simulink model "MdInOutChk"  (R2018b)
settings: Solver=FixedStepDiscrete  StartTime=0.0  StopTime=10.0  FixedStep=0.01  RelTol=1e-3
undefined symbols (not defined in the file or in its folder): MdRspLocal2
libraries: OutRspChkLib x20
(part 1 of 2)
settings Model: Creator=sn2xws  LastModifiedBy=sn2xws
settings DataIOCC: SaveFormat=StructureWithTime
settings OptimizationCC: DefaultParameterBehavior=Inlined  EnhancedBackFolding=on  PassReuseOutputArgsAs=Individual arguments  ZeroExternalMemoryAtStartup=off  ZeroInternalMemoryAtStartup=off  OptimizeBlockOrder=speed  DifferentSizesBufferReuse=on  OptimizationCustomize=off
settings DebuggingCC: ParameterTunabilityLossMsg=error
settings ModelReferenceCC: ModelReferenceNumInstancesAllowed=Single
settings SFSimCC: MATLABDynamicMemAlloc=off
settings RTWCC: SystemTargetFile=autosar.tlc  GenCodeOnly=on  TemplateMakefile=ert_default_tmf  Description=AUTOSAR  GenerateReport=on  IncludeHyperlinkInReport=on  LaunchReport=on  GenerateTraceInfo=on  GenerateTraceReport=on  GenerateTraceReportSl=on  GenerateTraceReportSf=on  GenerateTraceReportEml=on
settings CodeAppCC: ForceParamTrailComments=on  IgnoreCustomStorageClasses=off  OperatorAnnotations=on  SimulinkDataObjDesc=on  SFDataObjDesc=on  InsertBlockDesc=on
settings STFCustomTargetCC: TargetLangStandard=C99 (ISO)  MultiwordLength=256  ParMdlRefBuildCompliant=on  CompOptLevelCompliant=on  IncludeMdlTerminateFcn=off  CombineOutputUpdateFcns=on  SuppressErrorStatus=on  ERTCustomFileBanners=on  SupportNonFinite=off  SupportComplex=off  SupportContinuousTime=off  SupportNonInlinedSFcns=off  RemoveResetFunc=on  MATLABClassNameForMDSCustomization=Simulink.SoftwareTarget.ERTCustomization  AutosarCompliant=on  UseToolchainInfoCompliant=on  LookupTableObjectStructAxisOrder=2,1,3,4,...  LUTObjectStructOrderEvenSpacing=Size,Table,Breakpoints  SystemTargetFile=autosar.tlc
settings ERTTargetCC: TargetLangStandard=C99 (ISO)  ConcurrentExecutionCompliant=off  IncludeMdlTerminateFcn=off  SuppressErrorStatus=on  SupportNonFinite=off  SupportComplex=off  ModelStepFunctionPrototypeControlCompliant=off  CPPClassGenCompliant=off  AutosarCompliant=on  LookupTableObjectStructAxisOrder=2,1,3,4,...  LUTObjectStructOrderEvenSpacing=Size,Table,Breakpoints  InlinedParameterPlacement=NonHierarchical  ERTCustomFileTemplate=example_file_process.tlc

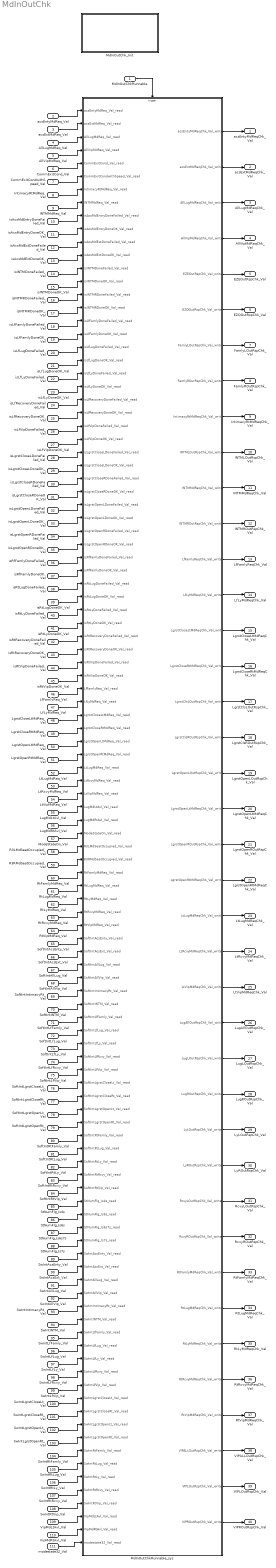
== system MdInOutChk ==
  MdInOutChkRunnable : Inport  SampleTime=0.01  OutputFunctionCall=on
  acsEntyMdReq_Val : Inport  Port=2  OutDataTypeStr=boolean  PortDimensions=1
  acsExtMdReq_Val : Inport  Port=3  OutDataTypeStr=boolean  PortDimensions=1
  AllLugMdReq_Val : Inport  Port=4  OutDataTypeStr=boolean  PortDimensions=1
  AllVipMdReq_Val : Inport  Port=5  OutDataTypeStr=boolean  PortDimensions=1
  CommExitCond_Val : Inport  Port=6  OutDataTypeStr=boolean  PortDimensions=1
  CommExitCondwithSpeed_Val : Inport  Port=7  OutDataTypeStr=boolean  PortDimensions=1
  IntimacyRtMdReq_Val : Inport  Port=8  OutDataTypeStr=boolean  PortDimensions=1
  INTMMdReq_Val : Inport  Port=9  OutDataTypeStr=boolean  PortDimensions=1
  isAcsMdEntryDoneFailed_Val : Inport  Port=10  OutDataTypeStr=boolean  PortDimensions=1
  isAcsMdEntryDoneOK_Val : Inport  Port=11  OutDataTypeStr=boolean  PortDimensions=1
  isAcsMdExtDoneFailed_Val : Inport  Port=12  OutDataTypeStr=boolean  PortDimensions=1
  isAcsMdExtDoneOK_Val : Inport  Port=13  OutDataTypeStr=boolean  PortDimensions=1
  isINTMDoneFailed_Val : Inport  Port=14  OutDataTypeStr=boolean  PortDimensions=1
  isINTMDoneOK_Val : Inport  Port=15  OutDataTypeStr=boolean  PortDimensions=1
  isINTMRDoneFailed_Val : Inport  Port=16  OutDataTypeStr=boolean  PortDimensions=1
  isINTMRDoneOK_Val : Inport  Port=17  OutDataTypeStr=boolean  PortDimensions=1
  isLfFamlyDoneFailed_Val : Inport  Port=18  OutDataTypeStr=boolean  PortDimensions=1
  isLfFamlyDoneOK_Val : Inport  Port=19  OutDataTypeStr=boolean  PortDimensions=1
  isLfLugDoneFailed_Val : Inport  Port=20  OutDataTypeStr=boolean  PortDimensions=1
  isLfLugDoneOK_Val : Inport  Port=21  OutDataTypeStr=boolean  PortDimensions=1
  isLfLyDoneFailed_Val : Inport  Port=22  OutDataTypeStr=boolean  PortDimensions=1
  isLfLyDoneOK_Val : Inport  Port=23  OutDataTypeStr=boolean  PortDimensions=1
  isLfRecoveryDoneFailed_Val : Inport  Port=24  OutDataTypeStr=boolean  PortDimensions=1
  isLfRecoveryDoneOK_Val : Inport  Port=25  OutDataTypeStr=boolean  PortDimensions=1
  isLfVipDoneFailed_Val : Inport  Port=26  OutDataTypeStr=boolean  PortDimensions=1
  isLfVipDoneOK_Val : Inport  Port=27  OutDataTypeStr=boolean  PortDimensions=1
  isLgrstCloseLDoneFailed_Val : Inport  Port=28  OutDataTypeStr=boolean  PortDimensions=1
  isLgrstCloseLDoneOK_Val : Inport  Port=29  OutDataTypeStr=boolean  PortDimensions=1
  isLgrstCloseRDoneFailed_Val : Inport  Port=30  OutDataTypeStr=boolean  PortDimensions=1
  isLgrstCloseRDoneOK_Val : Inport  Port=31  OutDataTypeStr=boolean  PortDimensions=1
  isLgrstOpenLDoneFailed_Val : Inport  Port=32  OutDataTypeStr=boolean  PortDimensions=1
  isLgrstOpenLDoneOK_Val : Inport  Port=33  OutDataTypeStr=boolean  PortDimensions=1
  isLgrstOpenRDoneFailed_Val : Inport  Port=34  OutDataTypeStr=boolean  PortDimensions=1
  isLgrstOpenRDoneOK_Val : Inport  Port=35  OutDataTypeStr=boolean  PortDimensions=1
  isRfFamlyDoneFailed_Val : Inport  Port=36  OutDataTypeStr=boolean  PortDimensions=1
  isRfFamlyDoneOK_Val : Inport  Port=37  OutDataTypeStr=boolean  PortDimensions=1
  isRtLugDoneFailed_Val : Inport  Port=38  OutDataTypeStr=boolean  PortDimensions=1
  isRtLugDoneOK_Val : Inport  Port=39  OutDataTypeStr=boolean  PortDimensions=1
  isRtLyDoneFailed_Val : Inport  Port=40  OutDataTypeStr=boolean  PortDimensions=1
  isRtLyDoneOK_Val : Inport  Port=41  OutDataTypeStr=boolean  PortDimensions=1
  isRtRecoveryDoneFailed_Val : Inport  Port=42  OutDataTypeStr=boolean  PortDimensions=1
  isRtRecoveryDoneOK_Val : Inport  Port=43  OutDataTypeStr=boolean  PortDimensions=1
  isRtVipDoneFailed_Val : Inport  Port=44  OutDataTypeStr=boolean  PortDimensions=1
  isRtVipDoneOK_Val : Inport  Port=45  OutDataTypeStr=boolean  PortDimensions=1
  LfFamlyReq_Val : Inport  Port=46  OutDataTypeStr=boolean  PortDimensions=1
  LfLyMdReq_Val : Inport  Port=47  OutDataTypeStr=boolean  PortDimensions=1
  LgrstCloseLtMdReq_Val : Inport  Port=48  OutDataTypeStr=boolean  PortDimensions=1
  LgrstCloseRtMdReq_Val : Inport  Port=49  OutDataTypeStr=boolean  PortDimensions=1
  LgrstOpenLtMdReq_Val : Inport  Port=50  OutDataTypeStr=boolean  PortDimensions=1
  LgrstOpenRtMdReq_Val : Inport  Port=51  OutDataTypeStr=boolean  PortDimensions=1
  LtLugMdReq_Val : Inport  Port=52  OutDataTypeStr=boolean  PortDimensions=1
  LtRcvyMdReq_Val : Inport  Port=53  OutDataTypeStr=boolean  PortDimensions=1
  LtVipMdReq_Val : Inport  Port=54  OutDataTypeStr=boolean  PortDimensions=1
  LugMdLtAvl_Val : Inport  Port=55  OutDataTypeStr=boolean  PortDimensions=1
  LugMdRtAvl_Val : Inport  Port=56  OutDataTypeStr=boolean  PortDimensions=1
  ModeStateOn_Val : Inport  Port=57  OutDataTypeStr=boolean  PortDimensions=1
  R3LMdSeatOccupied_Val : Inport  Port=58  OutDataTypeStr=boolean  PortDimensions=1
  R3RMdSeatOccupied_Val : Inport  Port=59  OutDataTypeStr=boolean  PortDimensions=1
  RtFamlyMdReq_Val : Inport  Port=60  OutDataTypeStr=boolean  PortDimensions=1
  RtLugMdReq_Val : Inport  Port=61  OutDataTypeStr=boolean  PortDimensions=1
  RtLyMdReq_Val : Inport  Port=62  OutDataTypeStr=boolean  PortDimensions=1
  RtRcvyMdReq_Val : Inport  Port=63  OutDataTypeStr=boolean  PortDimensions=1
  RtVipMdReq_Val : Inport  Port=64  OutDataTypeStr=boolean  PortDimensions=1
  SoftIntAcsEnty_Val : Inport  Port=65  OutDataTypeStr=IntEnable  PortDimensions=1
  SoftIntAcsExt_Val : Inport  Port=66  OutDataTypeStr=IntEnable  PortDimensions=1
  SoftIntAllLug_Val : Inport  Port=67  OutDataTypeStr=IntEnable  PortDimensions=1
  SoftIntAllVip_Val : Inport  Port=68  OutDataTypeStr=IntEnable  PortDimensions=1
  SoftIntIntimacyRt_Val : Inport  Port=69  OutDataTypeStr=IntEnable  PortDimensions=1
  SoftIntINTM_Val : Inport  Port=70  OutDataTypeStr=IntEnable  PortDimensions=1
  SoftIntLfFamly_Val : Inport  Port=71  OutDataTypeStr=IntEnable  PortDimensions=1
  SoftIntLfLug_Val : Inport  Port=72  OutDataTypeStr=IntEnable  PortDimensions=1
  SoftIntLfLy_Val : Inport  Port=73  OutDataTypeStr=IntEnable  PortDimensions=1
  SoftIntLfRcvy_Val : Inport  Port=74  OutDataTypeStr=IntEnable  PortDimensions=1
  SoftIntLfVip_Val : Inport  Port=75  OutDataTypeStr=IntEnable  PortDimensions=1
  SoftIntLgrstCloseLt_Val : Inport  Port=76  OutDataTypeStr=IntEnable  PortDimensions=1
  SoftIntLgrstCloseRt_Val : Inport  Port=77  OutDataTypeStr=IntEnable  PortDimensions=1
  SoftIntLgrstOpenLt_Val : Inport  Port=78  OutDataTypeStr=IntEnable  PortDimensions=1
  SoftIntLgrstOpenRt_Val : Inport  Port=79  OutDataTypeStr=IntEnable  PortDimensions=1
  SoftIntRtFamly_Val : Inport  Port=80  OutDataTypeStr=IntEnable  PortDimensions=1
  SoftIntRtLug_Val : Inport  Port=81  OutDataTypeStr=IntEnable  PortDimensions=1
  SoftIntRtLy_Val : Inport  Port=82  OutDataTypeStr=IntEnable  PortDimensions=1
  SoftIntRtRcvy_Val : Inport  Port=83  OutDataTypeStr=IntEnable  PortDimensions=1
  SoftIntRtVip_Val : Inport  Port=84  OutDataTypeStr=IntEnable  PortDimensions=1
  StNumFlg_Is4s : Inport  Port=85  OutDataTypeStr=boolean  PortDimensions=1
  StNumFlg_Is6s : Inport  Port=86  OutDataTypeStr=boolean  PortDimensions=1
  StNumFlg_Is6s7s : Inport  Port=87  OutDataTypeStr=boolean  PortDimensions=1
  StNumFlg_Is7s : Inport  Port=88  OutDataTypeStr=boolean  PortDimensions=1
  SwIntAcsEnty_Val : Inport  Port=89  OutDataTypeStr=IntEnable  PortDimensions=1
  SwIntAcsExt_Val : Inport  Port=90  OutDataTypeStr=IntEnable  PortDimensions=1
  SwIntAllLug_Val : Inport  Port=91  OutDataTypeStr=IntEnable  PortDimensions=1
  SwIntAllVip_Val : Inport  Port=92  OutDataTypeStr=IntEnable  PortDimensions=1
  SwIntIntimacyRt_Val : Inport  Port=93  OutDataTypeStr=IntEnable  PortDimensions=1
  SwIntINTM_Val : Inport  Port=94  OutDataTypeStr=IntEnable  PortDimensions=1
  SwIntLfFamly_Val : Inport  Port=95  OutDataTypeStr=IntEnable  PortDimensions=1
  SwIntLfLug_Val : Inport  Port=96  OutDataTypeStr=IntEnable  PortDimensions=1
  SwIntLfLy_Val : Inport  Port=97  OutDataTypeStr=IntEnable  PortDimensions=1
  SwIntLfRcvy_Val : Inport  Port=98  OutDataTypeStr=IntEnable  PortDimensions=1
  SwIntLfVip_Val : Inport  Port=99  OutDataTypeStr=IntEnable  PortDimensions=1
  SwIntLgrstCloseLt_Val : Inport  Port=100  OutDataTypeStr=IntEnable  PortDimensions=1
  SwIntLgrstCloseRt_Val : Inport  Port=101  OutDataTypeStr=IntEnable  PortDimensions=1
  SwIntLgrstOpenLt_Val : Inport  Port=102  OutDataTypeStr=IntEnable  PortDimensions=1
  SwIntLgrstOpenRt_Val : Inport  Port=103  OutDataTypeStr=IntEnable  PortDimensions=1
  SwIntRtFamly_Val : Inport  Port=104  OutDataTypeStr=IntEnable  PortDimensions=1
  SwIntRtLug_Val : Inport  Port=105  OutDataTypeStr=IntEnable  PortDimensions=1
  SwIntRtLy_Val : Inport  Port=106  OutDataTypeStr=IntEnable  PortDimensions=1
  SwIntRtRcvy_Val : Inport  Port=107  OutDataTypeStr=IntEnable  PortDimensions=1
  SwIntRtVip_Val : Inport  Port=108  OutDataTypeStr=IntEnable  PortDimensions=1
  VipMdLtAvl_Val : Inport  Port=109  OutDataTypeStr=boolean  PortDimensions=1
  VipMdRtAvl_Val : Inport  Port=110  OutDataTypeStr=boolean  PortDimensions=1
  modestate32_Val : Inport  Port=111  OutDataTypeStr=uint32  PortDimensions=1
  MdInOutChkRunnable_sys : Subsystem
  MdInOutChk_Init : Subsystem
  acsEntyMdReqChk_Val : Outport  OutDataTypeStr=boolean  PortDimensions=1
  acsExtMdReqChk_Val : Outport  Port=2  OutDataTypeStr=boolean  PortDimensions=1
  AllLugMdReqChk_Val : Outport  Port=3  OutDataTypeStr=boolean  PortDimensions=1
  AllVipMdReqChk_Val : Outport  Port=4  OutDataTypeStr=boolean  PortDimensions=1
  EZEOutRspChk_Val : Outport  Port=5  OutDataTypeStr=Enum: MdRspLocal2  PortDimensions=1
  EZQOutRspChk_Val : Outport  Port=6  OutDataTypeStr=Enum: MdRspLocal2  PortDimensions=1
  FamlyLOutRspChk_Val : Outport  Port=7  OutDataTypeStr=Enum: MdRspLocal2  PortDimensions=1
  FamlyROutRspChk_Val : Outport  Port=8  OutDataTypeStr=Enum: MdRspLocal2  PortDimensions=1
  IntimacyRtMdReqChk_Val : Outport  Port=9  OutDataTypeStr=boolean  PortDimensions=1
  INTMLOutRspChk_Val : Outport  Port=10  OutDataTypeStr=Enum: MdRspLocal2  PortDimensions=1
  INTMMdReqChk_Val : Outport  Port=11  OutDataTypeStr=boolean  PortDimensions=1
  INTMROutRspChk_Val : Outport  Port=12  OutDataTypeStr=Enum: MdRspLocal2  PortDimensions=1
  LfFamlyReqChk_Val : Outport  Port=13  OutDataTypeStr=boolean  PortDimensions=1
  LfLyMdReqChk_Val : Outport  Port=14  OutDataTypeStr=boolean  PortDimensions=1
  LgrstCloseLtMdReqChk_Val : Outport  Port=15  OutDataTypeStr=boolean  PortDimensions=1
  LgrstCloseRtMdReqChk_Val : Outport  Port=16  OutDataTypeStr=boolean  PortDimensions=1
  LgrstClsLOutRspChk_Val : Outport  Port=17  OutDataTypeStr=Enum: MdRspLocal2  PortDimensions=1
  LgrstClsROutRspChk_Val : Outport  Port=18  OutDataTypeStr=Enum: MdRspLocal2  PortDimensions=1
  LgrstOpenLOutRspChk_Val : Outport  Port=19  OutDataTypeStr=Enum: MdRspLocal2  PortDimensions=1
  LgrstOpenLtMdReqChk_Val : Outport  Port=20  OutDataTypeStr=boolean  PortDimensions=1
  LgrstOpenROutRspChk_Val : Outport  Port=21  OutDataTypeStr=Enum: MdRspLocal2  PortDimensions=1
  LgrstOpenRtMdReqChk_Val : Outport  Port=22  OutDataTypeStr=boolean  PortDimensions=1
  LtLugMdReqChk_Val : Outport  Port=23  OutDataTypeStr=boolean  PortDimensions=1
  LtRcvyMdReqChk_Val : Outport  Port=24  OutDataTypeStr=boolean  PortDimensions=1
  LtVipMdReqChk_Val : Outport  Port=25  OutDataTypeStr=boolean  PortDimensions=1
  LugAllOutRspChk_Val : Outport  Port=26  OutDataTypeStr=Enum: MdRspLocal2  PortDimensions=1
  LugLOutRspChk_Val : Outport  Port=27  OutDataTypeStr=Enum: MdRspLocal2  PortDimensions=1
  LugROutRspChk_Val : Outport  Port=28  OutDataTypeStr=Enum: MdRspLocal2  PortDimensions=1
  LyLOutRspChk_Val : Outport  Port=29  OutDataTypeStr=Enum: MdRspLocal2  PortDimensions=1
  LyROutRspChk_Val : Outport  Port=30  OutDataTypeStr=Enum: MdRspLocal2  PortDimensions=1
  RcvyLOutRspChk_Val : Outport  Port=31  OutDataTypeStr=Enum: MdRspLocal2  PortDimensions=1
  RcvyROutRspChk_Val : Outport  Port=32  OutDataTypeStr=Enum: MdRspLocal2  PortDimensions=1
  RtFamlyMdReqChk_Val : Outport  Port=33  OutDataTypeStr=boolean  PortDimensions=1
  RtLugMdReqChk_Val : Outport  Port=34  OutDataTypeStr=boolean  PortDimensions=1
  RtLyMdReqChk_Val : Outport  Port=35  OutDataTypeStr=boolean  PortDimensions=1
  RtRcvyMdReqChk_Val : Outport  Port=36  OutDataTypeStr=boolean  PortDimensions=1
  RtVipMdReqChk_Val : Outport  Port=37  OutDataTypeStr=boolean  PortDimensions=1
  VIPALLOutRspChk_Val : Outport  Port=38  OutDataTypeStr=Enum: MdRspLocal2  PortDimensions=1
  VIPLOutRspChk_Val : Outport  Port=39  OutDataTypeStr=Enum: MdRspLocal2  PortDimensions=1
  VIPROutRspChk_Val : Outport  Port=40  OutDataTypeStr=Enum: MdRspLocal2  PortDimensions=1
  wires:
  acsEntyMdReq_Val/1 -> MdInOutChkRunnable_sys/1(acsEntyMdReq_Val_read)
  acsExtMdReq_Val/1 -> MdInOutChkRunnable_sys/2(acsExtMdReq_Val_read)
  AllLugMdReq_Val/1 -> MdInOutChkRunnable_sys/3(AllLugMdReq_Val_read)
  AllVipMdReq_Val/1 -> MdInOutChkRunnable_sys/4(AllVipMdReq_Val_read)
  CommExitCond_Val/1 -> MdInOutChkRunnable_sys/5(CommExitCond_Val_read)
  CommExitCondwithSpeed_Val/1 -> MdInOutChkRunnable_sys/6(CommExitCondwithSpeed_Val_read)
  IntimacyRtMdReq_Val/1 -> MdInOutChkRunnable_sys/7(IntimacyRtMdReq_Val_read)
  INTMMdReq_Val/1 -> MdInOutChkRunnable_sys/8(INTMMdReq_Val_read)
  isAcsMdEntryDoneFailed_Val/1 -> MdInOutChkRunnable_sys/9(isAcsMdEntryDoneFailed_Val_read)
  isAcsMdEntryDoneOK_Val/1 -> MdInOutChkRunnable_sys/10(isAcsMdEntryDoneOK_Val_read)
  isAcsMdExtDoneFailed_Val/1 -> MdInOutChkRunnable_sys/11(isAcsMdExtDoneFailed_Val_read)
  isAcsMdExtDoneOK_Val/1 -> MdInOutChkRunnable_sys/12(isAcsMdExtDoneOK_Val_read)
  isINTMDoneFailed_Val/1 -> MdInOutChkRunnable_sys/13(isINTMDoneFailed_Val_read)
  isINTMDoneOK_Val/1 -> MdInOutChkRunnable_sys/14(isINTMDoneOK_Val_read)
  isINTMRDoneFailed_Val/1 -> MdInOutChkRunnable_sys/15(isINTMRDoneFailed_Val_read)
  isINTMRDoneOK_Val/1 -> MdInOutChkRunnable_sys/16(isINTMRDoneOK_Val_read)
  isLfFamlyDoneFailed_Val/1 -> MdInOutChkRunnable_sys/17(isLfFamlyDoneFailed_Val_read)
  isLfFamlyDoneOK_Val/1 -> MdInOutChkRunnable_sys/18(isLfFamlyDoneOK_Val_read)
  isLfLugDoneFailed_Val/1 -> MdInOutChkRunnable_sys/19(isLfLugDoneFailed_Val_read)
  isLfLugDoneOK_Val/1 -> MdInOutChkRunnable_sys/20(isLfLugDoneOK_Val_read)
  isLfLyDoneFailed_Val/1 -> MdInOutChkRunnable_sys/21(isLfLyDoneFailed_Val_read)
  isLfLyDoneOK_Val/1 -> MdInOutChkRunnable_sys/22(isLfLyDoneOK_Val_read)
  isLfRecoveryDoneFailed_Val/1 -> MdInOutChkRunnable_sys/23(isLfRecoveryDoneFailed_Val_read)
  isLfRecoveryDoneOK_Val/1 -> MdInOutChkRunnable_sys/24(isLfRecoveryDoneOK_Val_read)
  isLfVipDoneFailed_Val/1 -> MdInOutChkRunnable_sys/25(isLfVipDoneFailed_Val_read)
  isLfVipDoneOK_Val/1 -> MdInOutChkRunnable_sys/26(isLfVipDoneOK_Val_read)
  isLgrstCloseLDoneFailed_Val/1 -> MdInOutChkRunnable_sys/27(isLgrstCloseLDoneFailed_Val_read)
  isLgrstCloseLDoneOK_Val/1 -> MdInOutChkRunnable_sys/28(isLgrstCloseLDoneOK_Val_read)
  isLgrstCloseRDoneFailed_Val/1 -> MdInOutChkRunnable_sys/29(isLgrstCloseRDoneFailed_Val_read)
  isLgrstCloseRDoneOK_Val/1 -> MdInOutChkRunnable_sys/30(isLgrstCloseRDoneOK_Val_read)
  isLgrstOpenLDoneFailed_Val/1 -> MdInOutChkRunnable_sys/31(isLgrstOpenLDoneFailed_Val_read)
  isLgrstOpenLDoneOK_Val/1 -> MdInOutChkRunnable_sys/32(isLgrstOpenLDoneOK_Val_read)
  isLgrstOpenRDoneFailed_Val/1 -> MdInOutChkRunnable_sys/33(isLgrstOpenRDoneFailed_Val_read)
  isLgrstOpenRDoneOK_Val/1 -> MdInOutChkRunnable_sys/34(isLgrstOpenRDoneOK_Val_read)
  isRfFamlyDoneFailed_Val/1 -> MdInOutChkRunnable_sys/35(isRfFamlyDoneFailed_Val_read)
  isRfFamlyDoneOK_Val/1 -> MdInOutChkRunnable_sys/36(isRfFamlyDoneOK_Val_read)
  isRtLugDoneFailed_Val/1 -> MdInOutChkRunnable_sys/37(isRtLugDoneFailed_Val_read)
  isRtLugDoneOK_Val/1 -> MdInOutChkRunnable_sys/38(isRtLugDoneOK_Val_read)
  isRtLyDoneFailed_Val/1 -> MdInOutChkRunnable_sys/39(isRtLyDoneFailed_Val_read)
  isRtLyDoneOK_Val/1 -> MdInOutChkRunnable_sys/40(isRtLyDoneOK_Val_read)
  isRtRecoveryDoneFailed_Val/1 -> MdInOutChkRunnable_sys/41(isRtRecoveryDoneFailed_Val_read)
  isRtRecoveryDoneOK_Val/1 -> MdInOutChkRunnable_sys/42(isRtRecoveryDoneOK_Val_read)
  isRtVipDoneFailed_Val/1 -> MdInOutChkRunnable_sys/43(isRtVipDoneFailed_Val_read)
  isRtVipDoneOK_Val/1 -> MdInOutChkRunnable_sys/44(isRtVipDoneOK_Val_read)
  LfFamlyReq_Val/1 -> MdInOutChkRunnable_sys/45(LfFamlyReq_Val_read)
  LfLyMdReq_Val/1 -> MdInOutChkRunnable_sys/46(LfLyMdReq_Val_read)
  LgrstCloseLtMdReq_Val/1 -> MdInOutChkRunnable_sys/47(LgrstCloseLtMdReq_Val_read)
  LgrstCloseRtMdReq_Val/1 -> MdInOutChkRunnable_sys/48(LgrstCloseRtMdReq_Val_read)
  LgrstOpenLtMdReq_Val/1 -> MdInOutChkRunnable_sys/49(LgrstOpenLtMdReq_Val_read)
  LgrstOpenRtMdReq_Val/1 -> MdInOutChkRunnable_sys/50(LgrstOpenRtMdReq_Val_read)
  LtLugMdReq_Val/1 -> MdInOutChkRunnable_sys/51(LtLugMdReq_Val_read)
  LtRcvyMdReq_Val/1 -> MdInOutChkRunnable_sys/52(LtRcvyMdReq_Val_read)
  LtVipMdReq_Val/1 -> MdInOutChkRunnable_sys/53(LtVipMdReq_Val_read)
  LugMdLtAvl_Val/1 -> MdInOutChkRunnable_sys/54(LugMdLtAvl_Val_read)
  LugMdRtAvl_Val/1 -> MdInOutChkRunnable_sys/55(LugMdRtAvl_Val_read)
  ModeStateOn_Val/1 -> MdInOutChkRunnable_sys/56(ModeStateOn_Val_read)
  R3LMdSeatOccupied_Val/1 -> MdInOutChkRunnable_sys/57(R3LMdSeatOccupied_Val_read)
  R3RMdSeatOccupied_Val/1 -> MdInOutChkRunnable_sys/58(R3RMdSeatOccupied_Val_read)
  RtFamlyMdReq_Val/1 -> MdInOutChkRunnable_sys/59(RtFamlyMdReq_Val_read)
  RtLugMdReq_Val/1 -> MdInOutChkRunnable_sys/60(RtLugMdReq_Val_read)
  RtLyMdReq_Val/1 -> MdInOutChkRunnable_sys/61(RtLyMdReq_Val_read)
  RtRcvyMdReq_Val/1 -> MdInOutChkRunnable_sys/62(RtRcvyMdReq_Val_read)
  RtVipMdReq_Val/1 -> MdInOutChkRunnable_sys/63(RtVipMdReq_Val_read)
  SoftIntAcsEnty_Val/1 -> MdInOutChkRunnable_sys/64(SoftIntAcsEnty_Val_read)
  SoftIntAcsExt_Val/1 -> MdInOutChkRunnable_sys/65(SoftIntAcsExt_Val_read)
  SoftIntAllLug_Val/1 -> MdInOutChkRunnable_sys/66(SoftIntAllLug_Val_read)
  SoftIntAllVip_Val/1 -> MdInOutChkRunnable_sys/67(SoftIntAllVip_Val_read)
  SoftIntIntimacyRt_Val/1 -> MdInOutChkRunnable_sys/68(SoftIntIntimacyRt_Val_read)
  SoftIntINTM_Val/1 -> MdInOutChkRunnable_sys/69(SoftIntINTM_Val_read)
  SoftIntLfFamly_Val/1 -> MdInOutChkRunnable_sys/70(SoftIntLfFamly_Val_read)
  SoftIntLfLug_Val/1 -> MdInOutChkRunnable_sys/71(SoftIntLfLug_Val_read)
  SoftIntLfLy_Val/1 -> MdInOutChkRunnable_sys/72(SoftIntLfLy_Val_read)
  SoftIntLfRcvy_Val/1 -> MdInOutChkRunnable_sys/73(SoftIntLfRcvy_Val_read)
  SoftIntLfVip_Val/1 -> MdInOutChkRunnable_sys/74(SoftIntLfVip_Val_read)
  SoftIntLgrstCloseLt_Val/1 -> MdInOutChkRunnable_sys/75(SoftIntLgrstCloseLt_Val_read)
  SoftIntLgrstCloseRt_Val/1 -> MdInOutChkRunnable_sys/76(SoftIntLgrstCloseRt_Val_read)
  SoftIntLgrstOpenLt_Val/1 -> MdInOutChkRunnable_sys/77(SoftIntLgrstOpenLt_Val_read)
  SoftIntLgrstOpenRt_Val/1 -> MdInOutChkRunnable_sys/78(SoftIntLgrstOpenRt_Val_read)
  SoftIntRtFamly_Val/1 -> MdInOutChkRunnable_sys/79(SoftIntRtFamly_Val_read)
  SoftIntRtLug_Val/1 -> MdInOutChkRunnable_sys/80(SoftIntRtLug_Val_read)
  SoftIntRtLy_Val/1 -> MdInOutChkRunnable_sys/81(SoftIntRtLy_Val_read)
  SoftIntRtRcvy_Val/1 -> MdInOutChkRunnable_sys/82(SoftIntRtRcvy_Val_read)
  SoftIntRtVip_Val/1 -> MdInOutChkRunnable_sys/83(SoftIntRtVip_Val_read)
  StNumFlg_Is4s/1 -> MdInOutChkRunnable_sys/84(StNumFlg_Is4s_read)
  StNumFlg_Is6s/1 -> MdInOutChkRunnable_sys/85(StNumFlg_Is6s_read)
  StNumFlg_Is6s7s/1 -> MdInOutChkRunnable_sys/86(StNumFlg_Is6s7s_read)
  StNumFlg_Is7s/1 -> MdInOutChkRunnable_sys/87(StNumFlg_Is7s_read)
  SwIntAcsEnty_Val/1 -> MdInOutChkRunnable_sys/88(SwIntAcsEnty_Val_read)
  SwIntAcsExt_Val/1 -> MdInOutChkRunnable_sys/89(SwIntAcsExt_Val_read)
  SwIntAllLug_Val/1 -> MdInOutChkRunnable_sys/90(SwIntAllLug_Val_read)
  SwIntAllVip_Val/1 -> MdInOutChkRunnable_sys/91(SwIntAllVip_Val_read)
  SwIntIntimacyRt_Val/1 -> MdInOutChkRunnable_sys/92(SwIntIntimacyRt_Val_read)
  SwIntINTM_Val/1 -> MdInOutChkRunnable_sys/93(SwIntINTM_Val_read)
  SwIntLfFamly_Val/1 -> MdInOutChkRunnable_sys/94(SwIntLfFamly_Val_read)
  SwIntLfLug_Val/1 -> MdInOutChkRunnable_sys/95(SwIntLfLug_Val_read)
  SwIntLfLy_Val/1 -> MdInOutChkRunnable_sys/96(SwIntLfLy_Val_read)
  SwIntLfRcvy_Val/1 -> MdInOutChkRunnable_sys/97(SwIntLfRcvy_Val_read)
  SwIntLfVip_Val/1 -> MdInOutChkRunnable_sys/98(SwIntLfVip_Val_read)
  SwIntLgrstCloseLt_Val/1 -> MdInOutChkRunnable_sys/99(SwIntLgrstCloseLt_Val_read)
  SwIntLgrstCloseRt_Val/1 -> MdInOutChkRunnable_sys/100(SwIntLgrstCloseRt_Val_read)
  SwIntLgrstOpenLt_Val/1 -> MdInOutChkRunnable_sys/101(SwIntLgrstOpenLt_Val_read)
  SwIntLgrstOpenRt_Val/1 -> MdInOutChkRunnable_sys/102(SwIntLgrstOpenRt_Val_read)
  SwIntRtFamly_Val/1 -> MdInOutChkRunnable_sys/103(SwIntRtFamly_Val_read)
  SwIntRtLug_Val/1 -> MdInOutChkRunnable_sys/104(SwIntRtLug_Val_read)
  SwIntRtLy_Val/1 -> MdInOutChkRunnable_sys/105(SwIntRtLy_Val_read)
  SwIntRtRcvy_Val/1 -> MdInOutChkRunnable_sys/106(SwIntRtRcvy_Val_read)
  SwIntRtVip_Val/1 -> MdInOutChkRunnable_sys/107(SwIntRtVip_Val_read)
  VipMdLtAvl_Val/1 -> MdInOutChkRunnable_sys/108(VipMdLtAvl_Val_read)
  VipMdRtAvl_Val/1 -> MdInOutChkRunnable_sys/109(VipMdRtAvl_Val_read)
  MdInOutChkRunnable_sys/1(acsEntyMdReqChk_Val_write) -> acsEntyMdReqChk_Val/1
  MdInOutChkRunnable_sys/2(acsExtMdReqChk_Val_write) -> acsExtMdReqChk_Val/1
  MdInOutChkRunnable_sys/3(AllLugMdReqChk_Val_write) -> AllLugMdReqChk_Val/1
  MdInOutChkRunnable_sys/4(AllVipMdReqChk_Val_write) -> AllVipMdReqChk_Val/1
  MdInOutChkRunnable_sys/5(EZEOutRspChk_Val_write) -> EZEOutRspChk_Val/1
  MdInOutChkRunnable_sys/6(EZQOutRspChk_Val_write) -> EZQOutRspChk_Val/1
  MdInOutChkRunnable_sys/7(FamlyLOutRspChk_Val_write) -> FamlyLOutRspChk_Val/1
  MdInOutChkRunnable_sys/8(FamlyROutRspChk_Val_write) -> FamlyROutRspChk_Val/1
  MdInOutChkRunnable_sys/9(IntimacyRtMdReqChk_Val_write) -> IntimacyRtMdReqChk_Val/1
  MdInOutChkRunnable_sys/10(INTMLOutRspChk_Val_write) -> INTMLOutRspChk_Val/1
  MdInOutChkRunnable_sys/11(INTMMdReqChk_Val_write) -> INTMMdReqChk_Val/1
  MdInOutChkRunnable_sys/12(INTMROutRspChk_Val_write) -> INTMROutRspChk_Val/1
  MdInOutChkRunnable_sys/13(LfFamlyReqChk_Val_write) -> LfFamlyReqChk_Val/1
  MdInOutChkRunnable_sys/14(LfLyMdReqChk_Val_write) -> LfLyMdReqChk_Val/1
  MdInOutChkRunnable_sys/15(LgrstCloseLtMdReqChk_Val_write) -> LgrstCloseLtMdReqChk_Val/1
  MdInOutChkRunnable_sys/16(LgrstCloseRtMdReqChk_Val_write) -> LgrstCloseRtMdReqChk_Val/1
  MdInOutChkRunnable_sys/17(LgrstClsLOutRspChk_Val_write) -> LgrstClsLOutRspChk_Val/1
  MdInOutChkRunnable_sys/18(LgrstClsROutRspChk_Val_write) -> LgrstClsROutRspChk_Val/1
  MdInOutChkRunnable_sys/19(LgrstOpenLOutRspChk_Val_write) -> LgrstOpenLOutRspChk_Val/1
  MdInOutChkRunnable_sys/20(LgrstOpenLtMdReqChk_Val_write) -> LgrstOpenLtMdReqChk_Val/1
  MdInOutChkRunnable_sys/21(LgrstOpenROutRspChk_Val_write) -> LgrstOpenROutRspChk_Val/1
  MdInOutChkRunnable_sys/22(LgrstOpenRtMdReqChk_Val_write) -> LgrstOpenRtMdReqChk_Val/1
  MdInOutChkRunnable_sys/23(LtLugMdReqChk_Val_write) -> LtLugMdReqChk_Val/1
  MdInOutChkRunnable_sys/24(LtRcvyMdReqChk_Val_write) -> LtRcvyMdReqChk_Val/1
  MdInOutChkRunnable_sys/25(LtVipMdReqChk_Val_write) -> LtVipMdReqChk_Val/1
  MdInOutChkRunnable_sys/26(LugAllOutRspChk_Val_write) -> LugAllOutRspChk_Val/1
  MdInOutChkRunnable_sys/27(LugLOutRspChk_Val_write) -> LugLOutRspChk_Val/1
  MdInOutChkRunnable_sys/28(LugROutRspChk_Val_write) -> LugROutRspChk_Val/1
  MdInOutChkRunnable_sys/29(LyLOutRspChk_Val_write) -> LyLOutRspChk_Val/1
  MdInOutChkRunnable_sys/30(LyROutRspChk_Val_write) -> LyROutRspChk_Val/1
  MdInOutChkRunnable_sys/31(RcvyLOutRspChk_Val_write) -> RcvyLOutRspChk_Val/1
  MdInOutChkRunnable_sys/32(RcvyROutRspChk_Val_write) -> RcvyROutRspChk_Val/1
  MdInOutChkRunnable_sys/33(RtFamlyMdReqChk_Val_write) -> RtFamlyMdReqChk_Val/1
  MdInOutChkRunnable_sys/34(RtLugMdReqChk_Val_write) -> RtLugMdReqChk_Val/1
  MdInOutChkRunnable_sys/35(RtLyMdReqChk_Val_write) -> RtLyMdReqChk_Val/1
  MdInOutChkRunnable_sys/36(RtRcvyMdReqChk_Val_write) -> RtRcvyMdReqChk_Val/1
  MdInOutChkRunnable_sys/37(RtVipMdReqChk_Val_write) -> RtVipMdReqChk_Val/1
  MdInOutChkRunnable_sys/38(VIPALLOutRspChk_Val_write) -> VIPALLOutRspChk_Val/1
  MdInOutChkRunnable_sys/39(VIPLOutRspChk_Val_write) -> VIPLOutRspChk_Val/1
  MdInOutChkRunnable_sys/40(VIPROutRspChk_Val_write) -> VIPROutRspChk_Val/1
  MdInOutChkRunnable/1 -> MdInOutChkRunnable_sys/Trigger
  modestate32_Val/1 -> MdInOutChkRunnable_sys/110(modestate32_Val_read)

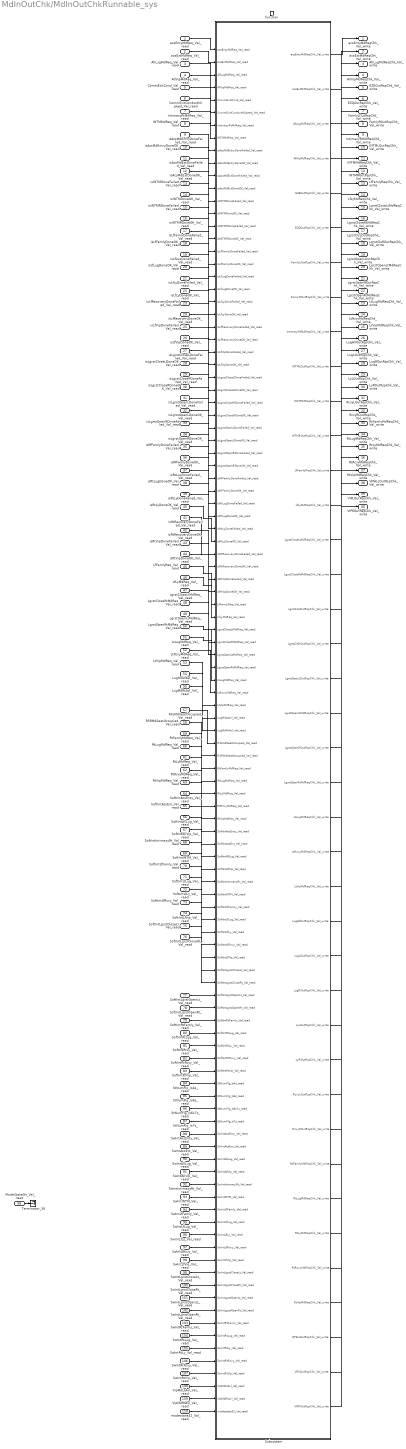
== system MdInOutChk/MdInOutChkRunnable_sys ==
  acsEntyMdReq_Val_read : Inport
  acsExtMdReq_Val_read : Inport  Port=2
  AllLugMdReq_Val_read : Inport  Port=3
  AllVipMdReq_Val_read : Inport  Port=4
  CommExitCond_Val_read : Inport  Port=5
  CommExitCondwithSpeed_Val_read : Inport  Port=6
  IntimacyRtMdReq_Val_read : Inport  Port=7
  INTMMdReq_Val_read : Inport  Port=8
  isAcsMdEntryDoneFailed_Val_read : Inport  Port=9
  isAcsMdEntryDoneOK_Val_read : Inport  Port=10
  isAcsMdExtDoneFailed_Val_read : Inport  Port=11
  isAcsMdExtDoneOK_Val_read : Inport  Port=12
  isINTMDoneFailed_Val_read : Inport  Port=13
  isINTMDoneOK_Val_read : Inport  Port=14
  isINTMRDoneFailed_Val_read : Inport  Port=15
  isINTMRDoneOK_Val_read : Inport  Port=16
  isLfFamlyDoneFailed_Val_read : Inport  Port=17
  isLfFamlyDoneOK_Val_read : Inport  Port=18
  isLfLugDoneFailed_Val_read : Inport  Port=19
  isLfLugDoneOK_Val_read : Inport  Port=20
  isLfLyDoneFailed_Val_read : Inport  Port=21
  isLfLyDoneOK_Val_read : Inport  Port=22
  isLfRecoveryDoneFailed_Val_read : Inport  Port=23
  isLfRecoveryDoneOK_Val_read : Inport  Port=24
  isLfVipDoneFailed_Val_read : Inport  Port=25
  isLfVipDoneOK_Val_read : Inport  Port=26
  isLgrstCloseLDoneFailed_Val_read : Inport  Port=27
  isLgrstCloseLDoneOK_Val_read : Inport  Port=28
  isLgrstCloseRDoneFailed_Val_read : Inport  Port=29
  isLgrstCloseRDoneOK_Val_read : Inport  Port=30
  isLgrstOpenLDoneFailed_Val_read : Inport  Port=31
  isLgrstOpenLDoneOK_Val_read : Inport  Port=32
  isLgrstOpenRDoneFailed_Val_read : Inport  Port=33
  isLgrstOpenRDoneOK_Val_read : Inport  Port=34
  isRfFamlyDoneFailed_Val_read : Inport  Port=35
  isRfFamlyDoneOK_Val_read : Inport  Port=36
  isRtLugDoneFailed_Val_read : Inport  Port=37
  isRtLugDoneOK_Val_read : Inport  Port=38
  isRtLyDoneFailed_Val_read : Inport  Port=39
  isRtLyDoneOK_Val_read : Inport  Port=40
  isRtRecoveryDoneFailed_Val_read : Inport  Port=41
  isRtRecoveryDoneOK_Val_read : Inport  Port=42
  isRtVipDoneFailed_Val_read : Inport  Port=43
  isRtVipDoneOK_Val_read : Inport  Port=44
  LfFamlyReq_Val_read : Inport  Port=45
  LfLyMdReq_Val_read : Inport  Port=46
  LgrstCloseLtMdReq_Val_read : Inport  Port=47
  LgrstCloseRtMdReq_Val_read : Inport  Port=48
  LgrstOpenLtMdReq_Val_read : Inport  Port=49
  LgrstOpenRtMdReq_Val_read : Inport  Port=50
  LtLugMdReq_Val_read : Inport  Port=51
  LtRcvyMdReq_Val_read : Inport  Port=52
  LtVipMdReq_Val_read : Inport  Port=53
  LugMdLtAvl_Val_read : Inport  Port=54
  LugMdRtAvl_Val_read : Inport  Port=55
  ModeStateOn_Val_read : Inport  Port=56
  R3LMdSeatOccupied_Val_read : Inport  Port=57
  R3RMdSeatOccupied_Val_read : Inport  Port=58
  RtFamlyMdReq_Val_read : Inport  Port=59
  RtLugMdReq_Val_read : Inport  Port=60
  RtLyMdReq_Val_read : Inport  Port=61
  RtRcvyMdReq_Val_read : Inport  Port=62
  RtVipMdReq_Val_read : Inport  Port=63
  SoftIntAcsEnty_Val_read : Inport  Port=64
  SoftIntAcsExt_Val_read : Inport  Port=65
  SoftIntAllLug_Val_read : Inport  Port=66
  SoftIntAllVip_Val_read : Inport  Port=67
  SoftIntIntimacyRt_Val_read : Inport  Port=68
  SoftIntINTM_Val_read : Inport  Port=69
  SoftIntLfFamly_Val_read : Inport  Port=70
  SoftIntLfLug_Val_read : Inport  Port=71
  SoftIntLfLy_Val_read : Inport  Port=72
  SoftIntLfRcvy_Val_read : Inport  Port=73
  SoftIntLfVip_Val_read : Inport  Port=74
  SoftIntLgrstCloseLt_Val_read : Inport  Port=75
  SoftIntLgrstCloseRt_Val_read : Inport  Port=76
  SoftIntLgrstOpenLt_Val_read : Inport  Port=77
  SoftIntLgrstOpenRt_Val_read : Inport  Port=78
  SoftIntRtFamly_Val_read : Inport  Port=79
  SoftIntRtLug_Val_read : Inport  Port=80
  SoftIntRtLy_Val_read : Inport  Port=81
  SoftIntRtRcvy_Val_read : Inport  Port=82
  SoftIntRtVip_Val_read : Inport  Port=83
  StNumFlg_Is4s_read : Inport  Port=84
  StNumFlg_Is6s_read : Inport  Port=85
  StNumFlg_Is6s7s_read : Inport  Port=86
  StNumFlg_Is7s_read : Inport  Port=87
  SwIntAcsEnty_Val_read : Inport  Port=88
  SwIntAcsExt_Val_read : Inport  Port=89
  SwIntAllLug_Val_read : Inport  Port=90
  SwIntAllVip_Val_read : Inport  Port=91
  SwIntIntimacyRt_Val_read : Inport  Port=92
  SwIntINTM_Val_read : Inport  Port=93
  SwIntLfFamly_Val_read : Inport  Port=94
  SwIntLfLug_Val_read : Inport  Port=95
  SwIntLfLy_Val_read : Inport  Port=96
  SwIntLfRcvy_Val_read : Inport  Port=97
  SwIntLfVip_Val_read : Inport  Port=98
  SwIntLgrstCloseLt_Val_read : Inport  Port=99
  SwIntLgrstCloseRt_Val_read : Inport  Port=100
  SwIntLgrstOpenLt_Val_read : Inport  Port=101
  SwIntLgrstOpenRt_Val_read : Inport  Port=102
  SwIntRtFamly_Val_read : Inport  Port=103
  SwIntRtLug_Val_read : Inport  Port=104
  SwIntRtLy_Val_read : Inport  Port=105
  SwIntRtRcvy_Val_read : Inport  Port=106
  SwIntRtVip_Val_read : Inport  Port=107
  VipMdLtAvl_Val_read : Inport  Port=108
  VipMdRtAvl_Val_read : Inport  Port=109
  modestate32_Val_read : Inport  Port=110
  function : TriggerPort  TriggerType=function-call  VariantControl=(inherit)  SampleTimeType=periodic  SampleTime=-1
  Subsystem : Subsystem
  Terminator_56 : Terminator
  acsEntyMdReqChk_Val_write : Outport
      settings: EnsureOutportIsVirtual=on
  acsExtMdReqChk_Val_write : Outport  Port=2
      settings: EnsureOutportIsVirtual=on
  AllLugMdReqChk_Val_write : Outport  Port=3
      settings: EnsureOutportIsVirtual=on
  AllVipMdReqChk_Val_write : Outport  Port=4
      settings: EnsureOutportIsVirtual=on
  EZEOutRspChk_Val_write : Outport  Port=5
      settings: EnsureOutportIsVirtual=on
  EZQOutRspChk_Val_write : Outport  Port=6
      settings: EnsureOutportIsVirtual=on
  FamlyLOutRspChk_Val_write : Outport  Port=7
      settings: EnsureOutportIsVirtual=on
  FamlyROutRspChk_Val_write : Outport  Port=8
      settings: EnsureOutportIsVirtual=on
  IntimacyRtMdReqChk_Val_write : Outport  Port=9
      settings: EnsureOutportIsVirtual=on
  INTMLOutRspChk_Val_write : Outport  Port=10
      settings: EnsureOutportIsVirtual=on
  INTMMdReqChk_Val_write : Outport  Port=11
      settings: EnsureOutportIsVirtual=on
  INTMROutRspChk_Val_write : Outport  Port=12
      settings: EnsureOutportIsVirtual=on
  LfFamlyReqChk_Val_write : Outport  Port=13
      settings: EnsureOutportIsVirtual=on
  LfLyMdReqChk_Val_write : Outport  Port=14
      settings: EnsureOutportIsVirtual=on
  LgrstCloseLtMdReqChk_Val_write : Outport  Port=15
      settings: EnsureOutportIsVirtual=on
  LgrstCloseRtMdReqChk_Val_write : Outport  Port=16
      settings: EnsureOutportIsVirtual=on
  LgrstClsLOutRspChk_Val_write : Outport  Port=17
      settings: EnsureOutportIsVirtual=on
  LgrstClsROutRspChk_Val_write : Outport  Port=18
      settings: EnsureOutportIsVirtual=on
  LgrstOpenLOutRspChk_Val_write : Outport  Port=19
      settings: EnsureOutportIsVirtual=on
  LgrstOpenLtMdReqChk_Val_write : Outport  Port=20
      settings: EnsureOutportIsVirtual=on
  LgrstOpenROutRspChk_Val_write : Outport  Port=21
      settings: EnsureOutportIsVirtual=on
  LgrstOpenRtMdReqChk_Val_write : Outport  Port=22
      settings: EnsureOutportIsVirtual=on
  LtLugMdReqChk_Val_write : Outport  Port=23
      settings: EnsureOutportIsVirtual=on
  LtRcvyMdReqChk_Val_write : Outport  Port=24
      settings: EnsureOutportIsVirtual=on
  LtVipMdReqChk_Val_write : Outport  Port=25
      settings: EnsureOutportIsVirtual=on
  LugAllOutRspChk_Val_write : Outport  Port=26
      settings: EnsureOutportIsVirtual=on
  LugLOutRspChk_Val_write : Outport  Port=27
      settings: EnsureOutportIsVirtual=on
  LugROutRspChk_Val_write : Outport  Port=28
      settings: EnsureOutportIsVirtual=on
  LyLOutRspChk_Val_write : Outport  Port=29
      settings: EnsureOutportIsVirtual=on
  LyROutRspChk_Val_write : Outport  Port=30
      settings: EnsureOutportIsVirtual=on
  RcvyLOutRspChk_Val_write : Outport  Port=31
      settings: EnsureOutportIsVirtual=on
  RcvyROutRspChk_Val_write : Outport  Port=32
      settings: EnsureOutportIsVirtual=on
  RtFamlyMdReqChk_Val_write : Outport  Port=33
      settings: EnsureOutportIsVirtual=on
  RtLugMdReqChk_Val_write : Outport  Port=34
      settings: EnsureOutportIsVirtual=on
  RtLyMdReqChk_Val_write : Outport  Port=35
      settings: EnsureOutportIsVirtual=on
  RtRcvyMdReqChk_Val_write : Outport  Port=36
      settings: EnsureOutportIsVirtual=on
  RtVipMdReqChk_Val_write : Outport  Port=37
      settings: EnsureOutportIsVirtual=on
  VIPALLOutRspChk_Val_write : Outport  Port=38
      settings: EnsureOutportIsVirtual=on
  VIPLOutRspChk_Val_write : Outport  Port=39
      settings: EnsureOutportIsVirtual=on
  VIPROutRspChk_Val_write : Outport  Port=40
      settings: EnsureOutportIsVirtual=on
  wires:
  ModeStateOn_Val_read/1 -> Terminator_56/1
  acsEntyMdReq_Val_read/1 -> Subsystem/1(acsEntyMdReq_Val_read)
  acsExtMdReq_Val_read/1 -> Subsystem/2(acsExtMdReq_Val_read)
  AllLugMdReq_Val_read/1 -> Subsystem/3(AllLugMdReq_Val_read)
  AllVipMdReq_Val_read/1 -> Subsystem/4(AllVipMdReq_Val_read)
  CommExitCond_Val_read/1 -> Subsystem/5(CommExitCond_Val_read)
  CommExitCondwithSpeed_Val_read/1 -> Subsystem/6(CommExitCondwithSpeed_Val_read)
  IntimacyRtMdReq_Val_read/1 -> Subsystem/7(IntimacyRtMdReq_Val_read)
  INTMMdReq_Val_read/1 -> Subsystem/8(INTMMdReq_Val_read)
  isAcsMdEntryDoneFailed_Val_read/1 -> Subsystem/9(isAcsMdEntryDoneFailed_Val_read)
  isAcsMdEntryDoneOK_Val_read/1 -> Subsystem/10(isAcsMdEntryDoneOK_Val_read)
  isAcsMdExtDoneFailed_Val_read/1 -> Subsystem/11(isAcsMdExtDoneFailed_Val_read)
  isAcsMdExtDoneOK_Val_read/1 -> Subsystem/12(isAcsMdExtDoneOK_Val_read)
  isINTMDoneFailed_Val_read/1 -> Subsystem/13(isINTMDoneFailed_Val_read)
  isINTMDoneOK_Val_read/1 -> Subsystem/14(isINTMDoneOK_Val_read)
  isINTMRDoneFailed_Val_read/1 -> Subsystem/15(isINTMRDoneFailed_Val_read)
  isINTMRDoneOK_Val_read/1 -> Subsystem/16(isINTMRDoneOK_Val_read)
  isLfFamlyDoneFailed_Val_read/1 -> Subsystem/17(isLfFamlyDoneFailed_Val_read)
  isLfFamlyDoneOK_Val_read/1 -> Subsystem/18(isLfFamlyDoneOK_Val_read)
  isLfLugDoneFailed_Val_read/1 -> Subsystem/19(isLfLugDoneFailed_Val_read)
  isLfLugDoneOK_Val_read/1 -> Subsystem/20(isLfLugDoneOK_Val_read)
  isLfLyDoneFailed_Val_read/1 -> Subsystem/21(isLfLyDoneFailed_Val_read)
  isLfLyDoneOK_Val_read/1 -> Subsystem/22(isLfLyDoneOK_Val_read)
  isLfRecoveryDoneFailed_Val_read/1 -> Subsystem/23(isLfRecoveryDoneFailed_Val_read)
  isLfRecoveryDoneOK_Val_read/1 -> Subsystem/24(isLfRecoveryDoneOK_Val_read)
  isLfVipDoneFailed_Val_read/1 -> Subsystem/25(isLfVipDoneFailed_Val_read)
  isLfVipDoneOK_Val_read/1 -> Subsystem/26(isLfVipDoneOK_Val_read)
  isLgrstCloseLDoneFailed_Val_read/1 -> Subsystem/27(isLgrstCloseLDoneFailed_Val_read)
  isLgrstCloseLDoneOK_Val_read/1 -> Subsystem/28(isLgrstCloseLDoneOK_Val_read)
  isLgrstCloseRDoneFailed_Val_read/1 -> Subsystem/29(isLgrstCloseRDoneFailed_Val_read)
  isLgrstCloseRDoneOK_Val_read/1 -> Subsystem/30(isLgrstCloseRDoneOK_Val_read)
  isLgrstOpenLDoneFailed_Val_read/1 -> Subsystem/31(isLgrstOpenLDoneFailed_Val_read)
  isLgrstOpenLDoneOK_Val_read/1 -> Subsystem/32(isLgrstOpenLDoneOK_Val_read)
  isLgrstOpenRDoneFailed_Val_read/1 -> Subsystem/33(isLgrstOpenRDoneFailed_Val_read)
  isLgrstOpenRDoneOK_Val_read/1 -> Subsystem/34(isLgrstOpenRDoneOK_Val_read)
  isRfFamlyDoneFailed_Val_read/1 -> Subsystem/35(isRfFamlyDoneFailed_Val_read)
  isRfFamlyDoneOK_Val_read/1 -> Subsystem/36(isRfFamlyDoneOK_Val_read)
  isRtLugDoneFailed_Val_read/1 -> Subsystem/37(isRtLugDoneFailed_Val_read)
  isRtLugDoneOK_Val_read/1 -> Subsystem/38(isRtLugDoneOK_Val_read)
  isRtLyDoneFailed_Val_read/1 -> Subsystem/39(isRtLyDoneFailed_Val_read)
  isRtLyDoneOK_Val_read/1 -> Subsystem/40(isRtLyDoneOK_Val_read)
  isRtRecoveryDoneFailed_Val_read/1 -> Subsystem/41(isRtRecoveryDoneFailed_Val_read)
  isRtRecoveryDoneOK_Val_read/1 -> Subsystem/42(isRtRecoveryDoneOK_Val_read)
  isRtVipDoneFailed_Val_read/1 -> Subsystem/43(isRtVipDoneFailed_Val_read)
  isRtVipDoneOK_Val_read/1 -> Subsystem/44(isRtVipDoneOK_Val_read)
  LfFamlyReq_Val_read/1 -> Subsystem/45(LfFamlyReq_Val_read)
  LfLyMdReq_Val_read/1 -> Subsystem/46(LfLyMdReq_Val_read)
  LgrstCloseLtMdReq_Val_read/1 -> Subsystem/47(LgrstCloseLtMdReq_Val_read)
  LgrstCloseRtMdReq_Val_read/1 -> Subsystem/48(LgrstCloseRtMdReq_Val_read)
  LgrstOpenLtMdReq_Val_read/1 -> Subsystem/49(LgrstOpenLtMdReq_Val_read)
  LgrstOpenRtMdReq_Val_read/1 -> Subsystem/50(LgrstOpenRtMdReq_Val_read)
  LtLugMdReq_Val_read/1 -> Subsystem/51(LtLugMdReq_Val_read)
  LtRcvyMdReq_Val_read/1 -> Subsystem/52(LtRcvyMdReq_Val_read)
  LtVipMdReq_Val_read/1 -> Subsystem/53(LtVipMdReq_Val_read)
  LugMdLtAvl_Val_read/1 -> Subsystem/54(LugMdLtAvl_Val_read)
  LugMdRtAvl_Val_read/1 -> Subsystem/55(LugMdRtAvl_Val_read)
  R3LMdSeatOccupied_Val_read/1 -> Subsystem/56(R3LMdSeatOccupied_Val_read)
  R3RMdSeatOccupied_Val_read/1 -> Subsystem/57(R3RMdSeatOccupied_Val_read)
  RtFamlyMdReq_Val_read/1 -> Subsystem/58(RtFamlyMdReq_Val_read)
  RtLugMdReq_Val_read/1 -> Subsystem/59(RtLugMdReq_Val_read)
  RtLyMdReq_Val_read/1 -> Subsystem/60(RtLyMdReq_Val_read)
  RtRcvyMdReq_Val_read/1 -> Subsystem/61(RtRcvyMdReq_Val_read)
  RtVipMdReq_Val_read/1 -> Subsystem/62(RtVipMdReq_Val_read)
  SoftIntAcsEnty_Val_read/1 -> Subsystem/63(SoftIntAcsEnty_Val_read)
  SoftIntAcsExt_Val_read/1 -> Subsystem/64(SoftIntAcsExt_Val_read)
  SoftIntAllLug_Val_read/1 -> Subsystem/65(SoftIntAllLug_Val_read)
  SoftIntAllVip_Val_read/1 -> Subsystem/66(SoftIntAllVip_Val_read)
  SoftIntIntimacyRt_Val_read/1 -> Subsystem/67(SoftIntIntimacyRt_Val_read)
  SoftIntINTM_Val_read/1 -> Subsystem/68(SoftIntINTM_Val_read)
  SoftIntLfFamly_Val_read/1 -> Subsystem/69(SoftIntLfFamly_Val_read)
  SoftIntLfLug_Val_read/1 -> Subsystem/70(SoftIntLfLug_Val_read)
  SoftIntLfLy_Val_read/1 -> Subsystem/71(SoftIntLfLy_Val_read)
  SoftIntLfRcvy_Val_read/1 -> Subsystem/72(SoftIntLfRcvy_Val_read)
  SoftIntLfVip_Val_read/1 -> Subsystem/73(SoftIntLfVip_Val_read)
  SoftIntLgrstCloseLt_Val_read/1 -> Subsystem/74(SoftIntLgrstCloseLt_Val_read)
  SoftIntLgrstCloseRt_Val_read/1 -> Subsystem/75(SoftIntLgrstCloseRt_Val_read)
  SoftIntLgrstOpenLt_Val_read/1 -> Subsystem/76(SoftIntLgrstOpenLt_Val_read)
  SoftIntLgrstOpenRt_Val_read/1 -> Subsystem/77(SoftIntLgrstOpenRt_Val_read)
  SoftIntRtFamly_Val_read/1 -> Subsystem/78(SoftIntRtFamly_Val_read)
  SoftIntRtLug_Val_read/1 -> Subsystem/79(SoftIntRtLug_Val_read)
  SoftIntRtLy_Val_read/1 -> Subsystem/80(SoftIntRtLy_Val_read)
  SoftIntRtRcvy_Val_read/1 -> Subsystem/81(SoftIntRtRcvy_Val_read)
  SoftIntRtVip_Val_read/1 -> Subsystem/82(SoftIntRtVip_Val_read)
  StNumFlg_Is4s_read/1 -> Subsystem/83(StNumFlg_Is4s_read)
  StNumFlg_Is6s_read/1 -> Subsystem/84(StNumFlg_Is6s_read)
  StNumFlg_Is6s7s_read/1 -> Subsystem/85(StNumFlg_Is6s7s_read)
  StNumFlg_Is7s_read/1 -> Subsystem/86(StNumFlg_Is7s_read)
  SwIntAcsEnty_Val_read/1 -> Subsystem/87(SwIntAcsEnty_Val_read)
  SwIntAcsExt_Val_read/1 -> Subsystem/88(SwIntAcsExt_Val_read)
  SwIntAllLug_Val_read/1 -> Subsystem/89(SwIntAllLug_Val_read)
  SwIntAllVip_Val_read/1 -> Subsystem/90(SwIntAllVip_Val_read)
  SwIntIntimacyRt_Val_read/1 -> Subsystem/91(SwIntIntimacyRt_Val_read)
  SwIntINTM_Val_read/1 -> Subsystem/92(SwIntINTM_Val_read)
  SwIntLfFamly_Val_read/1 -> Subsystem/93(SwIntLfFamly_Val_read)
  SwIntLfLug_Val_read/1 -> Subsystem/94(SwIntLfLug_Val_read)
  SwIntLfLy_Val_read/1 -> Subsystem/95(SwIntLfLy_Val_read)
  SwIntLfRcvy_Val_read/1 -> Subsystem/96(SwIntLfRcvy_Val_read)
  SwIntLfVip_Val_read/1 -> Subsystem/97(SwIntLfVip_Val_read)
  SwIntLgrstCloseLt_Val_read/1 -> Subsystem/98(SwIntLgrstCloseLt_Val_read)
  SwIntLgrstCloseRt_Val_read/1 -> Subsystem/99(SwIntLgrstCloseRt_Val_read)
  SwIntLgrstOpenLt_Val_read/1 -> Subsystem/100(SwIntLgrstOpenLt_Val_read)
  SwIntLgrstOpenRt_Val_read/1 -> Subsystem/101(SwIntLgrstOpenRt_Val_read)
  SwIntRtFamly_Val_read/1 -> Subsystem/102(SwIntRtFamly_Val_read)
  SwIntRtLug_Val_read/1 -> Subsystem/103(SwIntRtLug_Val_read)
  SwIntRtLy_Val_read/1 -> Subsystem/104(SwIntRtLy_Val_read)
  SwIntRtRcvy_Val_read/1 -> Subsystem/105(SwIntRtRcvy_Val_read)
  SwIntRtVip_Val_read/1 -> Subsystem/106(SwIntRtVip_Val_read)
  VipMdLtAvl_Val_read/1 -> Subsystem/107(VipMdLtAvl_Val_read)
  VipMdRtAvl_Val_read/1 -> Subsystem/108(VipMdRtAvl_Val_read)
  Subsystem/1(acsEntyMdReqChk_Val_write) -> acsEntyMdReqChk_Val_write/1
  Subsystem/2(acsExtMdReqChk_Val_write) -> acsExtMdReqChk_Val_write/1
  Subsystem/3(AllLugMdReqChk_Val_write) -> AllLugMdReqChk_Val_write/1
  Subsystem/4(AllVipMdReqChk_Val_write) -> AllVipMdReqChk_Val_write/1
  Subsystem/5(EZEOutRspChk_Val_write) -> EZEOutRspChk_Val_write/1
  Subsystem/6(EZQOutRspChk_Val_write) -> EZQOutRspChk_Val_write/1
  Subsystem/7(FamlyLOutRspChk_Val_write) -> FamlyLOutRspChk_Val_write/1
  Subsystem/8(FamlyROutRspChk_Val_write) -> FamlyROutRspChk_Val_write/1
  Subsystem/9(IntimacyRtMdReqChk_Val_write) -> IntimacyRtMdReqChk_Val_write/1
  Subsystem/10(INTMLOutRspChk_Val_write) -> INTMLOutRspChk_Val_write/1
  Subsystem/11(INTMMdReqChk_Val_write) -> INTMMdReqChk_Val_write/1
  Subsystem/12(INTMROutRspChk_Val_write) -> INTMROutRspChk_Val_write/1
  Subsystem/13(LfFamlyReqChk_Val_write) -> LfFamlyReqChk_Val_write/1
  Subsystem/14(LfLyMdReqChk_Val_write) -> LfLyMdReqChk_Val_write/1
  Subsystem/15(LgrstCloseLtMdReqChk_Val_write) -> LgrstCloseLtMdReqChk_Val_write/1
  Subsystem/16(LgrstCloseRtMdReqChk_Val_write) -> LgrstCloseRtMdReqChk_Val_write/1
  Subsystem/17(LgrstClsLOutRspChk_Val_write) -> LgrstClsLOutRspChk_Val_write/1
  Subsystem/18(LgrstClsROutRspChk_Val_write) -> LgrstClsROutRspChk_Val_write/1
  Subsystem/19(LgrstOpenLOutRspChk_Val_write) -> LgrstOpenLOutRspChk_Val_write/1
  Subsystem/20(LgrstOpenLtMdReqChk_Val_write) -> LgrstOpenLtMdReqChk_Val_write/1
  Subsystem/21(LgrstOpenROutRspChk_Val_write) -> LgrstOpenROutRspChk_Val_write/1
  Subsystem/22(LgrstOpenRtMdReqChk_Val_write) -> LgrstOpenRtMdReqChk_Val_write/1
  Subsystem/23(LtLugMdReqChk_Val_write) -> LtLugMdReqChk_Val_write/1
  Subsystem/24(LtRcvyMdReqChk_Val_write) -> LtRcvyMdReqChk_Val_write/1
  Subsystem/25(LtVipMdReqChk_Val_write) -> LtVipMdReqChk_Val_write/1
  Subsystem/26(LugAllOutRspChk_Val_write) -> LugAllOutRspChk_Val_write/1
  Subsystem/27(LugLOutRspChk_Val_write) -> LugLOutRspChk_Val_write/1
  Subsystem/28(LugROutRspChk_Val_write) -> LugROutRspChk_Val_write/1
  Subsystem/29(LyLOutRspChk_Val_write) -> LyLOutRspChk_Val_write/1
  Subsystem/30(LyROutRspChk_Val_write) -> LyROutRspChk_Val_write/1
  Subsystem/31(RcvyLOutRspChk_Val_write) -> RcvyLOutRspChk_Val_write/1
  Subsystem/32(RcvyROutRspChk_Val_write) -> RcvyROutRspChk_Val_write/1
  Subsystem/33(RtFamlyMdReqChk_Val_write) -> RtFamlyMdReqChk_Val_write/1
  Subsystem/34(RtLugMdReqChk_Val_write) -> RtLugMdReqChk_Val_write/1
  Subsystem/35(RtLyMdReqChk_Val_write) -> RtLyMdReqChk_Val_write/1
  Subsystem/36(RtRcvyMdReqChk_Val_write) -> RtRcvyMdReqChk_Val_write/1
  Subsystem/37(RtVipMdReqChk_Val_write) -> RtVipMdReqChk_Val_write/1
  Subsystem/38(VIPALLOutRspChk_Val_write) -> VIPALLOutRspChk_Val_write/1
  Subsystem/39(VIPLOutRspChk_Val_write) -> VIPLOutRspChk_Val_write/1
  Subsystem/40(VIPROutRspChk_Val_write) -> VIPROutRspChk_Val_write/1
  modestate32_Val_read/1 -> Subsystem/109(modestate32_Val_read)

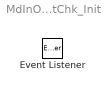
== system MdInOutChk/MdInOutChk_Init ==
  Event Listener : EventListener  EventName=reset
